simulink model "block190320_1"  (R2018a)
settings: Solver=FixedStepAuto  StartTime=0.0  StopTime=10.0  FixedStep=0.1  RelTol=1e-3
settings Model: Creator=Kenneth  LastModifiedBy=Kenneth

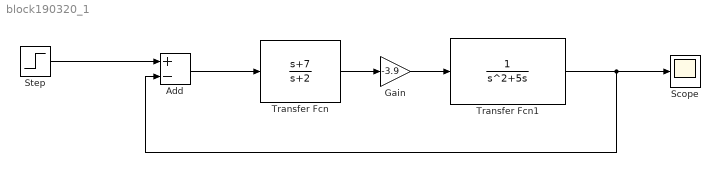
== system block190320_1 ==
  Add : Sum  Inputs=+-
  Gain : Gain  Gain=-3.9
  Scope : Scope
  Step : Step  SampleTime=0
  Transfer Fcn : TransferFcn  Numerator=[1,7]  Denominator=[1 2]
  Transfer Fcn1 : TransferFcn  Denominator=[1, 5, 0]
  wires:
  Step/1 -> Add/1
  Transfer Fcn1/1 -> Add/2, Scope/1
  Transfer Fcn/1 -> Gain/1
  Add/1 -> Transfer Fcn/1
  Gain/1 -> Transfer Fcn1/1
